simulink model "sar_temperature"  (R2021a)
settings: Solver=VariableStepAuto  StartTime=0.0  StopTime=50  RelTol=1e-3
libraries: pid_lib x1
settings Model: Creator=user  LastModifiedBy=user

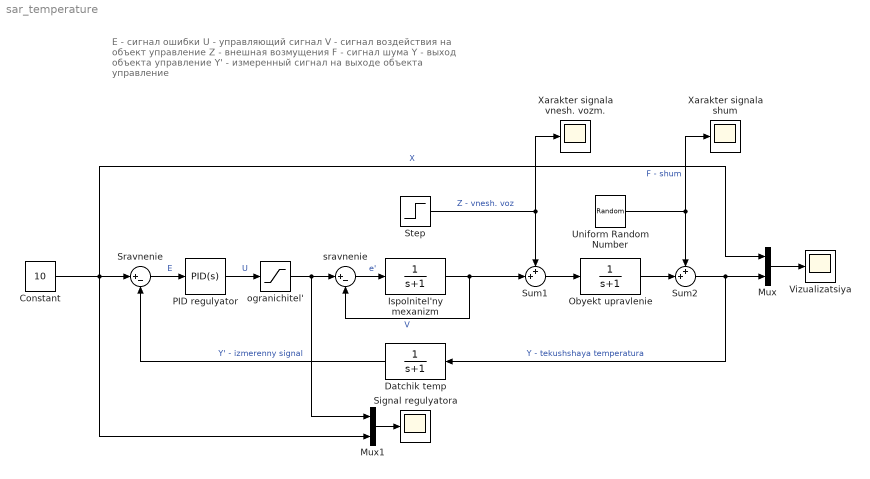
== system sar_temperature ==
  note: E - сигнал ошибки
      | U - управляющий сигнал
      | V - сигнал воздействия на объект управление
      | Z - внешная возмущения
      | F - сигнал шума
      | Y - выход объекта управление
      | Y' - измеренный сигнал на выходе объекта управление
  Constant : Constant  Value=10
  Datchik temp : TransferFcn  Denominator=[1 1]
  Ispolnitel'ny mexanizm : TransferFcn  Denominator=[1 1]
  Mux : Mux  Inputs=2
  Mux1 : Mux  Inputs=2
  Obyekt upravlenie : TransferFcn  Denominator=[1 1]
  PID regulyator : pid_lib/PID Controller  Controller=PID  Form=Parallel  TimeDomain=Continuous-time  UseExternalTs=off  SampleTime=-1  IntegratorMethod=Forward Euler  FilterMethod=Forward Euler  ControllerParametersSource=internal  P=0.0800591762648454  I=0.388180918773477  D=0  UseFilter=on  N=100  TunerSelectOption=Transfer Function Based (PID Tuner App)  InitialConditionSource=internal  InitialConditionForIntegrator=0  InitialConditionForFilter=0  DifferentiatorICPrevScaledInput=0  ExternalReset=none  TrackingMode=off  Kt=1  LimitOutput=off  SatLimitsSource=internal  UpperSaturationLimit=inf  LowerSaturationLimit=-inf  LinearizeAsGain=on  AntiWindupMode=none  Kb=1  POutMin=[]  POutMax=[]  IOutMin=[]  IOutMax=[]  DOutMin=[]  DOutMax=[]  NOutMin=[]  NOutMax=[]  SumOutMin=[]  SumOutMax=[]  SaturationOutMin=[]  SaturationOutMax=[]  PParamMin=[]  PParamMax=[]  IParamMin=[]  IParamMax=[]  DParamMin=[]  DParamMax=[]  NParamMin=[]  NParamMax=[]  KbParamMin=[]  KbParamMax=[]  KtParamMin=[]  KtParamMax=[]  KbOutMin=[]  KbOutMax=[]  KtOutMin=[]  KtOutMax=[]  IntegratorOutMin=[]  IntegratorOutMax=[]  FilterOutMin=[]  FilterOutMax=[]  SumI1OutMin=[]  SumI1OutMax=[]  SumI2OutMin=[]  SumI2OutMax=[]  SumI3OutMin=[]  SumI3OutMax=[]  SumI4OutMin=[]  SumI4OutMax=[]  SumDOutMin=[]  SumDOutMax=[]  DifferentiatorOutMin=[]  DifferentiatorOutMax=[]  FilterDiffOutCoefMin=[]  FilterDiffOutCoefMax=[]  ReciprocalOutMin=[]  ReciprocalOutMax=[]  SumDenOutMin=[]  SumDenOutMax=[]  SumNumOutMin=[]  SumNumOutMax=[]  DivideOutMin=[]  DivideOutMax=[]  UdiffTsProdOutMin=[]  UdiffTsProdOutMax=[]  NTsProdOutMin=[]  NTsProdOutMax=[]  UintegralTsProdOutMin=[]  UintegralTsProdOutMax=[]  UngainTsProdOutMin=[]  UngainTsProdOutMax=[]  IntegratorContinuousStateAttributes=''  IntegratorStateMustResolveToSignalObject=off  IntegratorRTWStateStorageClass=Auto  FilterContinuousStateAttributes=''  FilterStateMustResolveToSignalObject=off  FilterRTWStateStorageClass=Auto  ParallelPVariant=InternalParameters  IdealPVariant=Disabled  IVariant=InternalParameters  DVariant=InternalParameters  IntegratorVariant=Continuous  SatVariant=Disabled  AWVariant=Passthrough  PCopyVariant=Disabled  TRVariant=Disabled  FdbkBlocksVariant=Forward  IdealPFdbkVariant=Disabled  SatFdbkVariant=Disabled  DerivativeFilterVariant=ContFilter  NVariant=InternalParameters  NCopyVariant=Disabled  FilterICVariant=InternalICsFilter  IntegratorICVariant=InternalICs  ExternalResetVariant=Disabled  TRSumVariant=Passthrough  SumFdbkVariant=Disabled  SumVariant=Sum_PID  TsampFilterVariant=InternalTs  TsampNgainVariant=Passthrough  TsampIntegralVariant=Passthrough  ExternalSaturationOutDataTypeStr=Inherit: Same as second input
  Signal regulyatora : Scope
  Sravnenie : Sum  Inputs=|+-
  Step : Step  Time=25  After=3  SampleTime=0
  Sum1 : Sum  Inputs=++|
  Sum2 : Sum  Inputs=++|
  Uniform Random Number : UniformRandomNumber  Minimum=-0.5  Maximum=0.5  SampleTime=2
  Vizualizatsiya : Scope
  Xarakter signala shum : Scope
  Xarakter signala vnesh. vozm. : Scope
  ogranichitel' : Saturate  UpperLimit=100  LowerLimit=0
  sravnenie : Sum  Inputs=|+-
  wires:
  Constant/1 -> Mux1/2, Sravnenie/1, Mux/1  "X"
  Sravnenie/1 -> PID regulyator/1  "E"
  Mux/1 -> Vizualizatsiya/1
  Datchik temp/1 -> Sravnenie/2  "Y' - izmerenny signal"
  Sum2/1 -> Datchik temp/1, Mux/2  "Y - tekushshaya temperatura"
  PID regulyator/1 -> ogranichitel'/1  "U"
  Ispolnitel'ny mexanizm/1 -> Sum1/2, sravnenie/2  "V"
  Sum1/1 -> Obyekt upravlenie/1
  Obyekt upravlenie/1 -> Sum2/2
  Uniform Random Number/1 -> Xarakter signala shum/1, Sum2/1  "F - shum"
  Step/1 -> Xarakter signala vnesh. vozm./1, Sum1/1  "Z - vnesh. voz"
  ogranichitel'/1 -> Mux1/1, sravnenie/1
  sravnenie/1 -> Ispolnitel'ny mexanizm/1  "e'"
  Mux1/1 -> Signal regulyatora/1
